simulink model "V2X_Core_SRI_coding_rate_symbol"  (R2023b)
settings: Solver=ode23tb  StartTime=0.0  StopTime=50  MaxStep=1e-2  RelTol=1e-3  AbsTol=1e-3
StopFcn:
  | run('saving.m')
values from neighbouring files (symbols this model uses):
  b = 1.6    [a2024_v2x_matlab_6veh.m]
  m = 2000    [a2024_v2x_matlab_6veh.m]
  mEgo = 1500    [a2024_v2x_matlab_6veh.m]
  Mode = 1    [a2024_v2x_matlab_6veh.m]    (also in v2x_matlab.m; v2x_matlabV2.m; v2x_matlab_6veh.m; v2x_matlab_R.m)
  RefSpeed = 90/3.6    (= 25)    [v2x_matlabV2.m]    (also in v2x_matlab_R.m)
  RelDistThreshold = 300    [v2x_matlabV2.m]    (also in v2x_matlab_R.m)
  s = RandStream("dsfmt19937","Seed",15)    [v2x_matlab.m]
  sampleTime = 0.1    [a2024_v2x_matlab_6veh.m]    (also in v2x_matlab.m; v2x_matlabV2.m; v2x_matlab_6veh.m; v2x_matlab_R.m)
  waypoints = [egoWP(:,2) egoWP(:,1), zeroforwp]    [a2024_v2x_matlab_6veh.m]    (also in misc.m = data.data.ActorSpecifications(1,1).Waypoints(:,[1,2]); v2x_matlab.m = data.data.ActorSpecifications(1,1).Waypoints(:,[1,2]); v2x_matlabV2.m = [5 -1.6 0; v2x_matlab_R.m = [5 -1.6 0)
  ZeroActors = struct(     'ActorID',0,     'Position', [1000 1000 1000],      'Velocity', [0 0 0],      'Roll', 0,      'Pitch', 0,      'Yaw', 0,      'AngularVelocity', [0 0 0])    [v2x_matlabV2.m]    (also in v2x_matlab_R.m)
undefined symbols (not defined in the file or in its folder): Battery, Brakes, Control, DiscIntNeverNeededParam, doppler, Drivetrain, ElectricMotor, Env, FB_flag, Init, SNR_value_list, Vehicle, Wheels
libraries: simulink x45, commofdm x29, commdigbbndam3 x15, commchan3 x14, simulink_extras x13, commcnvcod2 x12, commdigbbndpm3 x11, commblkintrlv2 x10, dspmathops x6, sharedtransform x6, autolibutils x6, autolibsharedcoupling x4
(part 3 of 8)

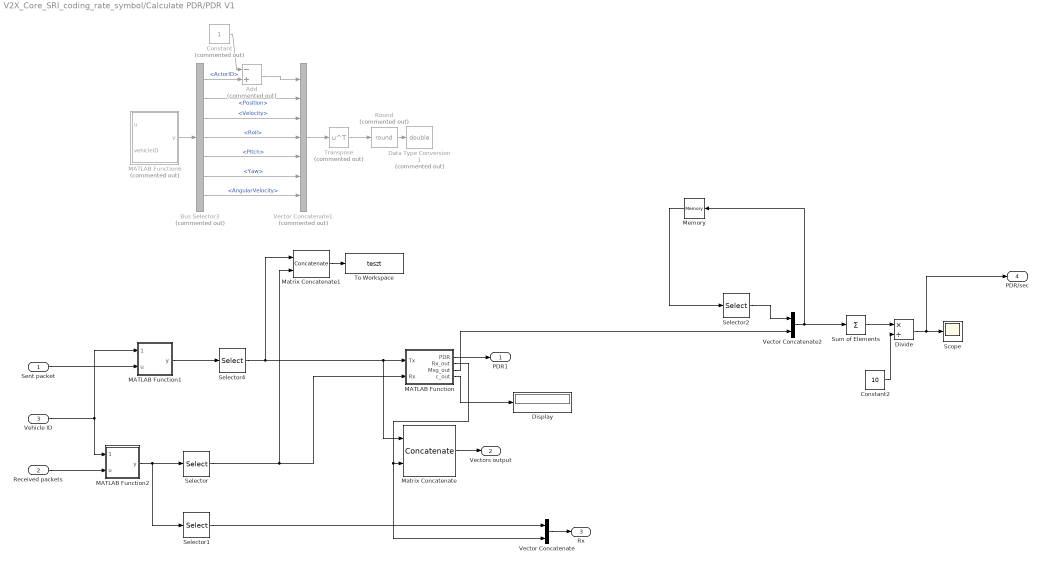
== system V2X_Core_SRI_coding_rate_symbol/Calculate PDR/PDR V1 ==
  Sent packet : Inport
  Received packets : Inport  Port=2
  Vehicle ID : Inport  Port=3
  Add : Sum  Commented=on  Inputs=-+
  Bus Selector3 : BusSelector  Commented=on  OutputSignals=ActorID,Position,Velocity,Roll,Pitch,Yaw,AngularVelocity
  Constant : Constant  Commented=on
  Constant2 : Constant  Value=10
  Data Type Conversion1 : DataTypeConversion  Commented=on  OutDataTypeStr=double  SaturateOnIntegerOverflow=off  RndMeth=Floor
  Display : Display
  Divide : Product  Inputs=*/
  MATLAB Function : MATLAB Function  TreatAsAtomicUnit=on
  MATLAB Function1 : MATLAB Function  TreatAsAtomicUnit=on
  MATLAB Function2 : MATLAB Function  TreatAsAtomicUnit=on
  MATLAB Function6 : MATLAB Function  Commented=on  TreatAsAtomicUnit=on
  Matrix Concatenate : Concatenate  Mode=Multidimensional array  ConcatenateDimension=2
  Matrix Concatenate1 : Concatenate  Mode=Multidimensional array  ConcatenateDimension=2
  Memory : Memory  InitialCondition=zeros(10,1)  InheritSampleTime=on
  Round : Rounding  Commented=on  Operator=round
  Scope : Scope
  Selector : Selector  InputPortWidth=15  IndexOptions=Starting index (dialog)  Indices=3  OutputSizes=13
  Selector1 : Selector  InputPortWidth=15  IndexOptions=Index vector (dialog)  Indices=[1 2]  OutputSizes=13
  Selector2 : Selector  InputPortWidth=10  IndexOptions=Index vector (dialog)  Indices=[2:10]  OutputSizes=1
  Selector4 : Selector  InputPortWidth=15  IndexOptions=Starting index (dialog)  Indices=3  OutputSizes=13
  Sum of Elements : Sum  Inputs=+
  To Workspace : ToWorkspace  VariableName=teszt  SampleTime=-1
  Transpose : Math  Commented=on  Operator=transpose
  Vector Concatenate : Concatenate
  Vector Concatenate1 : Concatenate  Commented=on  NumInputs=7
  Vector Concatenate2 : Concatenate
  PDR1 : Outport
  Vectors output : Outport  Port=2
  Rx : Outport  Port=3
  PDR/sec : Outport  Port=4
  wires:
  MATLAB Function2/1(y) -> Selector1/1, Selector/1
  Received packets/1 -> MATLAB Function2/2(u)
  Selector4/1 -> Matrix Concatenate1/1, Matrix Concatenate/1, MATLAB Function/1(Tx)
  MATLAB Function/1(PDR) -> PDR1/1
  Matrix Concatenate/1 -> Vectors output/1
  Selector/1 -> Matrix Concatenate1/2, MATLAB Function/2(Rx)
  Vehicle ID/1 -> MATLAB Function2/1(Vehicle_ID), MATLAB Function1/1(Vehicle_ID)
  MATLAB Function/2(Rx_out) -> Vector Concatenate/2, Matrix Concatenate/2
  Selector1/1 -> Vector Concatenate/1
  Vector Concatenate/1 -> Rx/1
  MATLAB Function/3(Msg_out) -> Vector Concatenate2/2
  Memory/1 -> Selector2/1
  Selector2/1 -> Vector Concatenate2/1
  Sum of Elements/1 -> Divide/1
  Constant2/1 -> Divide/2
  Divide/1 -> PDR/sec/1, Scope/1
  Vector Concatenate2/1 -> Memory/1, Sum of Elements/1
  Sent packet/1 -> MATLAB Function1/2(u)
  Add/1 -> Vector Concatenate1/1
  Bus Selector3/1 -> Add/2  "<ActorID>"
  Vector Concatenate1/1 -> Transpose/1
  Constant/1 -> Add/1
  Bus Selector3/5 -> Vector Concatenate1/5  "<Pitch>"
  Bus Selector3/2 -> Vector Concatenate1/2  "<Position>"
  Bus Selector3/7 -> Vector Concatenate1/7  "<AngularVelocity>"
  Transpose/1 -> Round/1
  Round/1 -> Data Type Conversion1/1
  Bus Selector3/4 -> Vector Concatenate1/4  "<Roll>"
  Bus Selector3/3 -> Vector Concatenate1/3  "<Velocity>"
  MATLAB Function6/1(y) -> Bus Selector3/1
  Bus Selector3/6 -> Vector Concatenate1/6  "<Yaw>"
  MATLAB Function1/1(y) -> Selector4/1
  MATLAB Function/4(c_out) -> Display/1
  Matrix Concatenate1/1 -> To Workspace/1

== system V2X_Core_SRI_coding_rate_symbol/Calculate PDR/PDR V2 ==
  Sent packet : Inport
  Received packets : Inport  Port=2
  Vehicle ID : Inport  Port=3
  Add : Sum  Commented=on  Inputs=-+
  Bus Selector3 : BusSelector  Commented=on  OutputSignals=ActorID,Position,Velocity,Roll,Pitch,Yaw,AngularVelocity
  Constant : Constant  Commented=on
  Constant2 : Constant  Value=10
  Data Type Conversion1 : DataTypeConversion  Commented=on  OutDataTypeStr=double  SaturateOnIntegerOverflow=off  RndMeth=Floor
  Divide : Product  Inputs=*/
  MATLAB Function : MATLAB Function  TreatAsAtomicUnit=on
  MATLAB Function1 : MATLAB Function  TreatAsAtomicUnit=on
  MATLAB Function2 : MATLAB Function  TreatAsAtomicUnit=on
  MATLAB Function6 : MATLAB Function  Commented=on  TreatAsAtomicUnit=on
  Matrix Concatenate : Concatenate  Mode=Multidimensional array  ConcatenateDimension=2
  Memory : Memory  InitialCondition=zeros(10,1)  InheritSampleTime=on
  Round : Rounding  Commented=on  Operator=round
  Scope : Scope
  Selector : Selector  InputPortWidth=15  IndexOptions=Starting index (dialog)  Indices=3  OutputSizes=13
  Selector1 : Selector  InputPortWidth=15  IndexOptions=Index vector (dialog)  Indices=[1 2]  OutputSizes=13
  Selector2 : Selector  InputPortWidth=10  IndexOptions=Index vector (dialog)  Indices=[2:10]  OutputSizes=1
  Selector4 : Selector  InputPortWidth=15  IndexOptions=Starting index (dialog)  Indices=3  OutputSizes=13
  Sum of Elements : Sum  Inputs=+
  Transpose : Math  Commented=on  Operator=transpose
  Vector Concatenate : Concatenate
  Vector Concatenate1 : Concatenate  Commented=on  NumInputs=7
  Vector Concatenate2 : Concatenate
  PDR2 : Outport
  Vectors output : Outport  Port=2
  Rx : Outport  Port=3
  PDR/sec : Outport  Port=4
  wires:
  MATLAB Function1/1(y) -> Selector4/1
  Bus Selector3/6 -> Vector Concatenate1/6  "<Yaw>"
  MATLAB Function6/1(y) -> Bus Selector3/1
  Bus Selector3/3 -> Vector Concatenate1/3  "<Velocity>"
  Bus Selector3/4 -> Vector Concatenate1/4  "<Roll>"
  Round/1 -> Data Type Conversion1/1
  Transpose/1 -> Round/1
  Bus Selector3/7 -> Vector Concatenate1/7  "<AngularVelocity>"
  Bus Selector3/2 -> Vector Concatenate1/2  "<Position>"
  Bus Selector3/5 -> Vector Concatenate1/5  "<Pitch>"
  Constant/1 -> Add/1
  Vector Concatenate1/1 -> Transpose/1
  Bus Selector3/1 -> Add/2  "<ActorID>"
  Add/1 -> Vector Concatenate1/1
  Sent packet/1 -> MATLAB Function1/2(u)
  Vector Concatenate2/1 -> Sum of Elements/1, Memory/1
  Divide/1 -> Scope/1, PDR/sec/1
  Constant2/1 -> Divide/2
  Sum of Elements/1 -> Divide/1
  Selector2/1 -> Vector Concatenate2/1
  Memory/1 -> Selector2/1
  MATLAB Function/3(Msg_out) -> Vector Concatenate2/2
  Vector Concatenate/1 -> Rx/1
  Selector1/1 -> Vector Concatenate/1
  MATLAB Function/2(Rx_out) -> Matrix Concatenate/2, Vector Concatenate/2
  Vehicle ID/1 -> MATLAB Function2/1(Vehicle_ID), MATLAB Function1/1(Vehicle_ID)
  Selector/1 -> MATLAB Function/2(Rx)
  Matrix Concatenate/1 -> Vectors output/1
  MATLAB Function/1(PDR) -> PDR2/1
  Selector4/1 -> MATLAB Function/1(Tx), Matrix Concatenate/1
  Received packets/1 -> MATLAB Function2/2(u)
  MATLAB Function2/1(y) -> Selector/1, Selector1/1

== system V2X_Core_SRI_coding_rate_symbol/Calculate PDR/PDR V3 ==
  Sent packet : Inport
  Received packets : Inport  Port=2
  Vehicle ID : Inport  Port=3
  Add : Sum  Commented=on  Inputs=-+
  Bus Selector3 : BusSelector  Commented=on  OutputSignals=ActorID,Position,Velocity,Roll,Pitch,Yaw,AngularVelocity
  Constant : Constant  Commented=on
  Constant2 : Constant  Value=10
  Data Type Conversion1 : DataTypeConversion  Commented=on  OutDataTypeStr=double  SaturateOnIntegerOverflow=off  RndMeth=Floor
  Divide : Product  Inputs=*/
  MATLAB Function : MATLAB Function  TreatAsAtomicUnit=on
  MATLAB Function1 : MATLAB Function  TreatAsAtomicUnit=on
  MATLAB Function2 : MATLAB Function  TreatAsAtomicUnit=on
  MATLAB Function6 : MATLAB Function  Commented=on  TreatAsAtomicUnit=on
  Matrix Concatenate : Concatenate  Mode=Multidimensional array  ConcatenateDimension=2
  Memory : Memory  InitialCondition=zeros(10,1)  InheritSampleTime=on
  Round : Rounding  Commented=on  Operator=round
  Scope : Scope
  Selector : Selector  InputPortWidth=15  IndexOptions=Starting index (dialog)  Indices=3  OutputSizes=13
  Selector1 : Selector  InputPortWidth=15  IndexOptions=Index vector (dialog)  Indices=[1 2]  OutputSizes=13
  Selector2 : Selector  InputPortWidth=10  IndexOptions=Index vector (dialog)  Indices=[2:10]  OutputSizes=1
  Selector4 : Selector  InputPortWidth=15  IndexOptions=Starting index (dialog)  Indices=3  OutputSizes=13
  Sum of Elements : Sum  Inputs=+
  Transpose : Math  Commented=on  Operator=transpose
  Vector Concatenate : Concatenate
  Vector Concatenate1 : Concatenate  Commented=on  NumInputs=7
  Vector Concatenate2 : Concatenate
  PDR3 : Outport
  Vectors output : Outport  Port=2
  Rx : Outport  Port=3
  PDR/sec : Outport  Port=4
  wires:
  MATLAB Function2/1(y) -> Selector1/1, Selector/1
  Received packets/1 -> MATLAB Function2/2(u)
  Selector4/1 -> Matrix Concatenate/1, MATLAB Function/1(Tx)
  MATLAB Function/1(PDR) -> PDR3/1
  Matrix Concatenate/1 -> Vectors output/1
  Selector/1 -> MATLAB Function/2(Rx)
  Vehicle ID/1 -> MATLAB Function1/1(Vehicle_ID), MATLAB Function2/1(Vehicle_ID)
  MATLAB Function/2(Rx_out) -> Vector Concatenate/2, Matrix Concatenate/2
  Selector1/1 -> Vector Concatenate/1
  Vector Concatenate/1 -> Rx/1
  MATLAB Function/3(Msg_out) -> Vector Concatenate2/2
  Memory/1 -> Selector2/1
  Selector2/1 -> Vector Concatenate2/1
  Sum of Elements/1 -> Divide/1
  Constant2/1 -> Divide/2
  Divide/1 -> PDR/sec/1, Scope/1
  Vector Concatenate2/1 -> Memory/1, Sum of Elements/1
  Sent packet/1 -> MATLAB Function1/2(u)
  Add/1 -> Vector Concatenate1/1
  Bus Selector3/1 -> Add/2  "<ActorID>"
  Vector Concatenate1/1 -> Transpose/1
  Constant/1 -> Add/1
  Bus Selector3/5 -> Vector Concatenate1/5  "<Pitch>"
  Bus Selector3/2 -> Vector Concatenate1/2  "<Position>"
  Bus Selector3/7 -> Vector Concatenate1/7  "<AngularVelocity>"
  Transpose/1 -> Round/1
  Round/1 -> Data Type Conversion1/1
  Bus Selector3/4 -> Vector Concatenate1/4  "<Roll>"
  Bus Selector3/3 -> Vector Concatenate1/3  "<Velocity>"
  MATLAB Function6/1(y) -> Bus Selector3/1
  Bus Selector3/6 -> Vector Concatenate1/6  "<Yaw>"
  MATLAB Function1/1(y) -> Selector4/1

== system V2X_Core_SRI_coding_rate_symbol/Calculate PDR/PDR V4 ==
  Sent packet : Inport
  Received packets : Inport  Port=2
  Vehicle ID : Inport  Port=3
  Add : Sum  Commented=on  Inputs=-+
  Bus Selector3 : BusSelector  Commented=on  OutputSignals=ActorID,Position,Velocity,Roll,Pitch,Yaw,AngularVelocity
  Constant : Constant  Commented=on
  Constant2 : Constant  Value=10
  Data Type Conversion1 : DataTypeConversion  Commented=on  OutDataTypeStr=double  SaturateOnIntegerOverflow=off  RndMeth=Floor
  Divide : Product  Inputs=*/
  MATLAB Function : MATLAB Function  TreatAsAtomicUnit=on
  MATLAB Function1 : MATLAB Function  TreatAsAtomicUnit=on
  MATLAB Function2 : MATLAB Function  TreatAsAtomicUnit=on
  MATLAB Function6 : MATLAB Function  Commented=on  TreatAsAtomicUnit=on
  Matrix Concatenate : Concatenate  Mode=Multidimensional array  ConcatenateDimension=2
  Memory : Memory  InitialCondition=zeros(10,1)  InheritSampleTime=on
  Round : Rounding  Commented=on  Operator=round
  Scope : Scope
  Selector : Selector  InputPortWidth=15  IndexOptions=Starting index (dialog)  Indices=3  OutputSizes=13
  Selector1 : Selector  InputPortWidth=15  IndexOptions=Index vector (dialog)  Indices=[1 2]  OutputSizes=13
  Selector2 : Selector  InputPortWidth=10  IndexOptions=Index vector (dialog)  Indices=[2:10]  OutputSizes=1
  Selector4 : Selector  InputPortWidth=15  IndexOptions=Starting index (dialog)  Indices=3  OutputSizes=13
  Sum of Elements : Sum  Inputs=+
  Transpose : Math  Commented=on  Operator=transpose
  Vector Concatenate : Concatenate
  Vector Concatenate1 : Concatenate  Commented=on  NumInputs=7
  Vector Concatenate2 : Concatenate
  PDR1 : Outport
  Vectors output : Outport  Port=2
  Rx : Outport  Port=3
  PDR/sec : Outport  Port=4
  wires:
  MATLAB Function1/1(y) -> Selector4/1
  Bus Selector3/6 -> Vector Concatenate1/6  "<Yaw>"
  MATLAB Function6/1(y) -> Bus Selector3/1
  Bus Selector3/3 -> Vector Concatenate1/3  "<Velocity>"
  Bus Selector3/4 -> Vector Concatenate1/4  "<Roll>"
  Round/1 -> Data Type Conversion1/1
  Transpose/1 -> Round/1
  Bus Selector3/7 -> Vector Concatenate1/7  "<AngularVelocity>"
  Bus Selector3/2 -> Vector Concatenate1/2  "<Position>"
  Bus Selector3/5 -> Vector Concatenate1/5  "<Pitch>"
  Constant/1 -> Add/1
  Vector Concatenate1/1 -> Transpose/1
  Bus Selector3/1 -> Add/2  "<ActorID>"
  Add/1 -> Vector Concatenate1/1
  Sent packet/1 -> MATLAB Function1/2(u)
  Vector Concatenate2/1 -> Sum of Elements/1, Memory/1
  Divide/1 -> Scope/1, PDR/sec/1
  Constant2/1 -> Divide/2
  Sum of Elements/1 -> Divide/1
  Selector2/1 -> Vector Concatenate2/1
  Memory/1 -> Selector2/1
  MATLAB Function/3(Msg_out) -> Vector Concatenate2/2
  Vector Concatenate/1 -> Rx/1
  Selector1/1 -> Vector Concatenate/1
  MATLAB Function/2(Rx_out) -> Matrix Concatenate/2, Vector Concatenate/2
  Vehicle ID/1 -> MATLAB Function2/1(Vehicle_ID), MATLAB Function1/1(Vehicle_ID)
  Selector/1 -> MATLAB Function/2(Rx)
  Matrix Concatenate/1 -> Vectors output/1
  MATLAB Function/1(PDR) -> PDR1/1
  Selector4/1 -> MATLAB Function/1(Tx), Matrix Concatenate/1
  Received packets/1 -> MATLAB Function2/2(u)
  MATLAB Function2/1(y) -> Selector/1, Selector1/1

== system V2X_Core_SRI_coding_rate_symbol/Calculate PDR/PDR V5 ==
  Sent packet : Inport
  Received packets : Inport  Port=2
  Vehicle ID : Inport  Port=3
  Add : Sum  Commented=on  Inputs=-+
  Bus Selector3 : BusSelector  Commented=on  OutputSignals=ActorID,Position,Velocity,Roll,Pitch,Yaw,AngularVelocity
  Constant : Constant  Commented=on
  Constant2 : Constant  Value=10
  Data Type Conversion1 : DataTypeConversion  Commented=on  OutDataTypeStr=double  SaturateOnIntegerOverflow=off  RndMeth=Floor
  Divide : Product  Inputs=*/
  MATLAB Function : MATLAB Function  TreatAsAtomicUnit=on
  MATLAB Function1 : MATLAB Function  TreatAsAtomicUnit=on
  MATLAB Function2 : MATLAB Function  TreatAsAtomicUnit=on
  MATLAB Function6 : MATLAB Function  Commented=on  TreatAsAtomicUnit=on
  Matrix Concatenate : Concatenate  Mode=Multidimensional array  ConcatenateDimension=2
  Memory : Memory  InitialCondition=zeros(10,1)  InheritSampleTime=on
  Round : Rounding  Commented=on  Operator=round
  Scope : Scope
  Selector : Selector  InputPortWidth=15  IndexOptions=Starting index (dialog)  Indices=3  OutputSizes=13
  Selector1 : Selector  InputPortWidth=15  IndexOptions=Index vector (dialog)  Indices=[1 2]  OutputSizes=13
  Selector2 : Selector  InputPortWidth=10  IndexOptions=Index vector (dialog)  Indices=[2:10]  OutputSizes=1
  Selector4 : Selector  InputPortWidth=15  IndexOptions=Starting index (dialog)  Indices=3  OutputSizes=13
  Sum of Elements : Sum  Inputs=+
  Transpose : Math  Commented=on  Operator=transpose
  Vector Concatenate : Concatenate
  Vector Concatenate1 : Concatenate  Commented=on  NumInputs=7
  Vector Concatenate2 : Concatenate
  PDR1 : Outport
  Vectors output : Outport  Port=2
  Rx : Outport  Port=3
  PDR/sec : Outport  Port=4
  wires:
  MATLAB Function2/1(y) -> Selector1/1, Selector/1
  Received packets/1 -> MATLAB Function2/2(u)
  Selector4/1 -> Matrix Concatenate/1, MATLAB Function/1(Tx)
  MATLAB Function/1(PDR) -> PDR1/1
  Matrix Concatenate/1 -> Vectors output/1
  Selector/1 -> MATLAB Function/2(Rx)
  Vehicle ID/1 -> MATLAB Function1/1(Vehicle_ID), MATLAB Function2/1(Vehicle_ID)
  MATLAB Function/2(Rx_out) -> Vector Concatenate/2, Matrix Concatenate/2
  Selector1/1 -> Vector Concatenate/1
  Vector Concatenate/1 -> Rx/1
  MATLAB Function/3(Msg_out) -> Vector Concatenate2/2
  Memory/1 -> Selector2/1
  Selector2/1 -> Vector Concatenate2/1
  Sum of Elements/1 -> Divide/1
  Constant2/1 -> Divide/2
  Divide/1 -> PDR/sec/1, Scope/1
  Vector Concatenate2/1 -> Memory/1, Sum of Elements/1
  Sent packet/1 -> MATLAB Function1/2(u)
  Add/1 -> Vector Concatenate1/1
  Bus Selector3/1 -> Add/2  "<ActorID>"
  Vector Concatenate1/1 -> Transpose/1
  Constant/1 -> Add/1
  Bus Selector3/5 -> Vector Concatenate1/5  "<Pitch>"
  Bus Selector3/2 -> Vector Concatenate1/2  "<Position>"
  Bus Selector3/7 -> Vector Concatenate1/7  "<AngularVelocity>"
  Transpose/1 -> Round/1
  Round/1 -> Data Type Conversion1/1
  Bus Selector3/4 -> Vector Concatenate1/4  "<Roll>"
  Bus Selector3/3 -> Vector Concatenate1/3  "<Velocity>"
  MATLAB Function6/1(y) -> Bus Selector3/1
  Bus Selector3/6 -> Vector Concatenate1/6  "<Yaw>"
  MATLAB Function1/1(y) -> Selector4/1

== system V2X_Core_SRI_coding_rate_symbol/Calculate PDR/PDR V6 ==
  Sent packet : Inport
  Received packets : Inport  Port=2
  Vehicle ID : Inport  Port=3
  Add : Sum  Commented=on  Inputs=-+
  Bus Selector3 : BusSelector  Commented=on  OutputSignals=ActorID,Position,Velocity,Roll,Pitch,Yaw,AngularVelocity
  Constant : Constant  Commented=on
  Constant2 : Constant  Value=10
  Data Type Conversion1 : DataTypeConversion  Commented=on  OutDataTypeStr=double  SaturateOnIntegerOverflow=off  RndMeth=Floor
  Divide : Product  Inputs=*/
  MATLAB Function : MATLAB Function  TreatAsAtomicUnit=on
  MATLAB Function1 : MATLAB Function  TreatAsAtomicUnit=on
  MATLAB Function2 : MATLAB Function  TreatAsAtomicUnit=on
  MATLAB Function6 : MATLAB Function  Commented=on  TreatAsAtomicUnit=on
  Matrix Concatenate : Concatenate  Mode=Multidimensional array  ConcatenateDimension=2
  Memory : Memory  InitialCondition=zeros(10,1)  InheritSampleTime=on
  Round : Rounding  Commented=on  Operator=round
  Scope : Scope
  Selector : Selector  InputPortWidth=15  IndexOptions=Starting index (dialog)  Indices=3  OutputSizes=13
  Selector1 : Selector  InputPortWidth=15  IndexOptions=Index vector (dialog)  Indices=[1 2]  OutputSizes=13
  Selector2 : Selector  InputPortWidth=10  IndexOptions=Index vector (dialog)  Indices=[2:10]  OutputSizes=1
  Selector4 : Selector  InputPortWidth=15  IndexOptions=Starting index (dialog)  Indices=3  OutputSizes=13
  Sum of Elements : Sum  Inputs=+
  Transpose : Math  Commented=on  Operator=transpose
  Vector Concatenate : Concatenate
  Vector Concatenate1 : Concatenate  Commented=on  NumInputs=7
  Vector Concatenate2 : Concatenate
  PDR1 : Outport
  Vectors output : Outport  Port=2
  Rx : Outport  Port=3
  PDR/sec : Outport  Port=4
  wires:
  MATLAB Function1/1(y) -> Selector4/1
  Bus Selector3/6 -> Vector Concatenate1/6  "<Yaw>"
  MATLAB Function6/1(y) -> Bus Selector3/1
  Bus Selector3/3 -> Vector Concatenate1/3  "<Velocity>"
  Bus Selector3/4 -> Vector Concatenate1/4  "<Roll>"
  Round/1 -> Data Type Conversion1/1
  Transpose/1 -> Round/1
  Bus Selector3/7 -> Vector Concatenate1/7  "<AngularVelocity>"
  Bus Selector3/2 -> Vector Concatenate1/2  "<Position>"
  Bus Selector3/5 -> Vector Concatenate1/5  "<Pitch>"
  Constant/1 -> Add/1
  Vector Concatenate1/1 -> Transpose/1
  Bus Selector3/1 -> Add/2  "<ActorID>"
  Add/1 -> Vector Concatenate1/1
  Sent packet/1 -> MATLAB Function1/2(u)
  Vector Concatenate2/1 -> Sum of Elements/1, Memory/1
  Divide/1 -> Scope/1, PDR/sec/1
  Constant2/1 -> Divide/2
  Sum of Elements/1 -> Divide/1
  Selector2/1 -> Vector Concatenate2/1
  Memory/1 -> Selector2/1
  MATLAB Function/3(Msg_out) -> Vector Concatenate2/2
  Vector Concatenate/1 -> Rx/1
  Selector1/1 -> Vector Concatenate/1
  MATLAB Function/2(Rx_out) -> Matrix Concatenate/2, Vector Concatenate/2
  Vehicle ID/1 -> MATLAB Function2/1(Vehicle_ID), MATLAB Function1/1(Vehicle_ID)
  Selector/1 -> MATLAB Function/2(Rx)
  Matrix Concatenate/1 -> Vectors output/1
  MATLAB Function/1(PDR) -> PDR1/1
  Selector4/1 -> MATLAB Function/1(Tx), Matrix Concatenate/1
  Received packets/1 -> MATLAB Function2/2(u)
  MATLAB Function2/1(y) -> Selector/1, Selector1/1

== system V2X_Core_SRI_coding_rate_symbol/DSRC/Queue ==
  Actors : Inport
  Bus Selector : BusSelector  OutputSignals=Actor1,Actor2,Actor3,Actor4,Actor5,Actor6
  Counter Limited : simulink/Sources/Counter Limited  uplimit=4  tsamp=0.01
  Merge : Merge  Inputs=6
  Scope1 : Scope
  Switch Case : SwitchCase  CaseConditions={0,1,2,3,4,5}  ShowDefaultCase=off
  Switch Case Action Subsystem : Subsystem  TreatAsAtomicUnit=on
  Switch Case Action Subsystem1 : Subsystem  TreatAsAtomicUnit=on
  Switch Case Action Subsystem2 : Subsystem  TreatAsAtomicUnit=on
  Switch Case Action Subsystem3 : Subsystem  TreatAsAtomicUnit=on
  Switch Case Action Subsystem4 : Subsystem  TreatAsAtomicUnit=on
  Switch Case Action Subsystem5 : Subsystem  TreatAsAtomicUnit=on
  Actor : Outport
  wires:
  Switch Case/4 -> Switch Case Action Subsystem3/Action
  Switch Case Action Subsystem5/1(Out1) -> Merge/6
  Counter Limited/1 -> Switch Case/1, Scope1/1  "Control"
  Switch Case/2 -> Switch Case Action Subsystem1/Action
  Switch Case Action Subsystem3/1(Out1) -> Merge/4
  Switch Case Action Subsystem4/1(Out1) -> Merge/5
  Switch Case/1 -> Switch Case Action Subsystem/Action
  Switch Case/6 -> Switch Case Action Subsystem5/Action
  Switch Case Action Subsystem2/1(Out1) -> Merge/3
  Switch Case/3 -> Switch Case Action Subsystem2/Action
  Switch Case/5 -> Switch Case Action Subsystem4/Action
  Switch Case Action Subsystem1/1(Out1) -> Merge/2
  Bus Selector/2 -> Switch Case Action Subsystem1/1(Actor1)  "<Actor2>"
  Bus Selector/3 -> Switch Case Action Subsystem2/1(In1)  "<Actor3>"
  Bus Selector/4 -> Switch Case Action Subsystem3/1(In1)  "<Actor4>"
  Bus Selector/5 -> Switch Case Action Subsystem4/1(In1)  "<Actor5>"
  Bus Selector/6 -> Switch Case Action Subsystem5/1(In1)  "<Actor6>"
  Actors/1 -> Bus Selector/1
  Bus Selector/1 -> Switch Case Action Subsystem/1(Actor1)  "<Actor1>"
  Merge/1 -> Actor/1
  Switch Case Action Subsystem/1(Actor) -> Merge/1

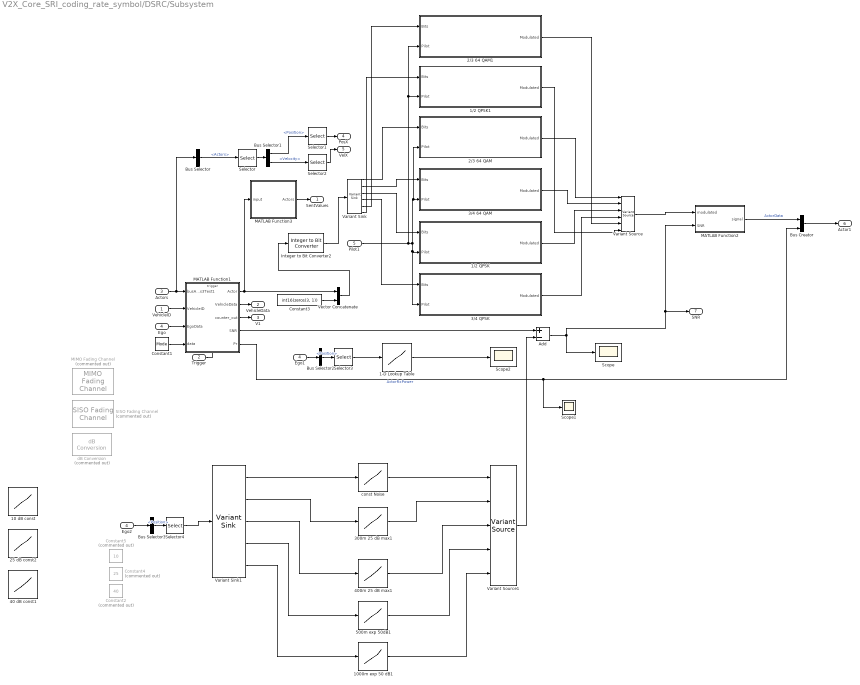
== system V2X_Core_SRI_coding_rate_symbol/DSRC/Subsystem ==
  VehicleID : Inport
  Trigger : Inport  Port=2
  Actors : Inport  Port=3
  Ego : Inport  Port=4
  Pilot1 : Inport  Port=5
  " 10 dB const" : Lookup_n-D  NumberOfTableDimensions=1  BreakpointsForDimension1=[0 100 200 300 400 500 600 700 800 900 1000]  Table=[10 10 10 10 10 10 10 10 10 10 10]  InternalRulePriority=Speed  RndMeth=Simplest
  " 25 dB const2" : Lookup_n-D  NumberOfTableDimensions=1  BreakpointsForDimension1=[0 100 200 300 400 500 600 700 800 900 1000]  Table=[25 25 25 25 25 25 25 25 25 25 25]  InternalRulePriority=Speed  RndMeth=Simplest
  " 40 dB const1" : Lookup_n-D  NumberOfTableDimensions=1  BreakpointsForDimension1=[0 100 200 300 400 500 600 700 800 900 1000]  Table=[40 40 40 40 40 40 40 40 40 40 40]  InternalRulePriority=Speed  RndMeth=Simplest
  1-D Lookup Table : Lookup_n-D  NumberOfTableDimensions=1  BreakpointsForDimension1=[0 100 200 300 400 500 600 700 800 900 1000]  Table=[5 10 15 20 15 10 5 0 0 0 0]  InternalRulePriority=Speed  RndMeth=Simplest
  1/2 QPSK : Subsystem  TreatAsAtomicUnit=on
  1/2 QPSK1 : Subsystem  TreatAsAtomicUnit=on
  1000m exp 50 dB1 : Lookup_n-D  NumberOfTableDimensions=1  BreakpointsForDimension1=[0;100;200;300;400;500;600;700;800;900;1000;2000]  Table=[1;1;1.58;2.51;3.98;6.31;10;15.85;25.12;39.81;50;50]  InternalRulePriority=Speed  RndMeth=Simplest
  2/3 64 QAM : Subsystem  TreatAsAtomicUnit=on
  2/3 64 QAM1 : Subsystem  TreatAsAtomicUnit=on
  3/4 64 QAM : Subsystem  TreatAsAtomicUnit=on
  3/4 QPSK : Subsystem  TreatAsAtomicUnit=on
  300m 25 dB max1 : Lookup_n-D  NumberOfTableDimensions=1  BreakpointsForDimension1=[0 100 200 300 400 500 600 700 800 900 1000]  Table=[10 15 20 25 20 15 10 5 0 0 0]  InternalRulePriority=Speed  RndMeth=Simplest
  400m 25 dB max1 : Lookup_n-D  NumberOfTableDimensions=1  BreakpointsForDimension1=[0 100 200 300 400 500 600 700 800 900 1000]  Table=[5 10 15 20 25 20 15 10 5 0 0]  InternalRulePriority=Speed  RndMeth=Simplest
  500m exp 50dB1 : Lookup_n-D  NumberOfTableDimensions=1  BreakpointsForDimension1=[0;100;200;300;400;500;600;700;800;900;1000;2000]  Table=[1;1;1.58;2.51;3.98;6.31;10;15.85;25.12;39.81;50;50]  InternalRulePriority=Speed  RndMeth=Simplest
  Add : Sum  Inputs=+-
  Bus Creator : BusCreator  Inputs=2
  Bus Selector : BusSelector  OutputSignals=Actors
  Bus Selector1 : BusSelector  OutputSignals=Position,Velocity
  Bus Selector2 : BusSelector  OutputSignals=Position
  Bus Selector3 : BusSelector  OutputSignals=Position
  Constant1 : Constant  Value=Mode
  Constant2 : Constant  Commented=on  Value=40
  Constant3 : Constant  Value=int16(zeros(3, 1))
  Constant4 : Constant  Commented=on  Value=25
  Constant5 : Constant  Commented=on  Value=10
  Ego1 : InportShadow  Port=4
  Ego2 : InportShadow  Port=4
  Integer to Bit Converter2 : simulink/Logic and Bit Operations/Integer to Bit Converter  nbits=16  signedInputValues=Signed  bitOrder=MSB first  outDtype=int16
  MATLAB Function1 : MATLAB Function  TreatAsAtomicUnit=on
  MATLAB Function2 : MATLAB Function  TreatAsAtomicUnit=on
  MATLAB Function3 : MATLAB Function  TreatAsAtomicUnit=on  SystemSampleTime=0.01
  MIMO Fading Channel : commchan3/MIMO Fading Channel  Commented=on  InheritSampleRate=on  SampleRate=1  PathDelays=0  AveragePathGains=0  NormalizePathGains=on  FadingDistribution=Rayleigh  KFactor=3  DirectPathDopplerShift=0  DirectPathInitialPhase=0  MaximumDopplerShift=0.001  DopplerSpectrum=doppler('Jakes')  SpatialCorrelationSpecification=None  SpatialCorrelationMatrix=[1 0 0 0; 0 1 0 0; 0 0 1 0; 0 0 0 1]  NumTransmitAntennas=1  NumReceiveAntennas=1  TransmitCorrelationMatrix=[1 0; 0 1]  ReceiveCorrelationMatrix=[1 0; 0 1]  AntennaSelection=Off  NormalizeChannelOutputs=on  PathGainsOutputPort=off  SimulateUsing=Interpreted execution  FadingTechnique=Filtered Gaussian noise  NumSinusoids=48  InitialTimeSource=Property  InitialTime=0  RandomStream=mt19937ar with seed  Seed=73  Visualization=Off  AntennaPairsToDisplay=[ 1, 1 ]  PathsForDopplerDisplay=1  SamplesToDisplay=25%
  SISO Fading Channel : commchan3/SISO Fading Channel  Commented=on  InheritSampleRate=off  SampleRate=5.9e9  PathDelays=0  AveragePathGains=0  NormalizePathGains=on  FadingDistribution=Rayleigh  KFactor=3  DirectPathDopplerShift=0  DirectPathInitialPhase=0  MaximumDopplerShift=0.001  DopplerSpectrum=doppler('Jakes')  RandomStream=mt19937ar with seed  Seed=73  PathGainsOutputPort=off  ChannelFilterDelayOutputPort=off  SimulateUsing=Interpreted execution  Visualization=Off  PathsForDopplerDisplay=1  SamplesToDisplay=25%
  Scope : Scope
  Scope1 : Scope
  Scope2 : Scope
  Selector : Selector  InputPortWidth=1  IndexOptions=Index vector (dialog)  Indices=1  OutputSizes=1
  Selector1 : Selector  InputPortWidth=3  IndexOptions=Index vector (dialog)  Indices=1  OutputSizes=1
  Selector2 : Selector  InputPortWidth=3  IndexOptions=Index vector (dialog)  Indices=1  OutputSizes=1
  Selector3 : Selector  InputPortWidth=3  IndexOptions=Index vector (dialog)  Indices=[1]  OutputSizes=1
  Selector4 : Selector  InputPortWidth=3  IndexOptions=Index vector (dialog)  Indices=[1]  OutputSizes=1
  Variant Sink : VariantSink
  Variant Sink1 : VariantSink
  Variant Source : VariantSource
  Variant Source1 : VariantSource
  Vector Concatenate : Concatenate
  const Noise : Lookup_n-D  NumberOfTableDimensions=1  BreakpointsForDimension1=[0 100 200 300 400 500 600 700 800 900 1000]  Table=SNR_value_list  InternalRulePriority=Speed  RndMeth=Simplest
  dB Conversion : dspmathops/dB Conversion  Commented=on  dBtype=dB  intype=Amplitude  R=1  fuzz=off
      settings: LibrarySourceBlock=commutil2/dB Conversion
  SentValues : Outport
  VehicleData : Outport  Port=2
  V1 : Outport  Port=3
  PosX : Outport  Port=4
  VelX : Outport  Port=5
  Actor1 : Outport  Port=6
  SNR : Outport  Port=7
  wires:
  MATLAB Function1/1(Actor) -> MATLAB Function3/1(input), Vector Concatenate/1
  Ego/1 -> MATLAB Function1/3(EgoData)
  Actors/1 -> Bus Selector/1, MATLAB Function1/1(busActors3Test1)
  VehicleID/1 -> MATLAB Function1/2(VehicleID)
  MATLAB Function1/2(VehicleData) -> VehicleData/1
  MATLAB Function1/3(counter_out) -> V1/1
  Trigger/1 -> MATLAB Function1/Trigger
  MATLAB Function1/5(Pr) -> Scope1/1, Bus Creator/2  "ActorRxPower"
  MATLAB Function1/4(SNR) -> Add/1
  Add/1 -> SNR/1, MATLAB Function2/2(SNR), Scope/1
  Selector1/1 -> PosX/1
  Bus Selector/1 -> Selector/1  "<Actors>"
  Selector/1 -> Bus Selector1/1
  Bus Selector1/1 -> Selector1/1  "<Position>"
  Bus Selector1/2 -> Selector2/1  "<Velocity>"
  Selector2/1 -> VelX/1
  Variant Sink/4 -> 3/4 QPSK/1(Bits)
  Pilot1/1 -> 1/2 QPSK1/2(Pilot), 2/3 64 QAM1/2(Pilot), 3/4 QPSK/2(Pilot), 1/2 QPSK/2(Pilot), 2/3 64 QAM/2(Pilot), 3/4 64 QAM/2(Pilot)
  Integer to Bit Converter2/1 -> Variant Sink/1
  3/4 QPSK/1(Modulated) -> Variant Source/4
  3/4 64 QAM/1(Modulated) -> Variant Source/2
  Variant Sink/2 -> 3/4 64 QAM/1(Bits)
  Bus Creator/1 -> Actor1/1
  MATLAB Function3/1(Actors) -> SentValues/1
  Constant1/1 -> MATLAB Function1/4(data)
  1-D Lookup Table/1 -> Scope2/1
  Constant3/1 -> Vector Concatenate/2
  Vector Concatenate/1 -> Integer to Bit Converter2/1
  Variant Source/1 -> MATLAB Function2/1(modulated)
  MATLAB Function2/1(signal) -> Bus Creator/1  "ActorData"
  Variant Sink/3 -> 1/2 QPSK/1(Bits)
  Variant Sink/1 -> 2/3 64 QAM/1(Bits)
  1/2 QPSK/1(Modulated) -> Variant Source/3
  2/3 64 QAM/1(Modulated) -> Variant Source/1
  Ego1/1 -> Bus Selector2/1
  Bus Selector2/1 -> Selector3/1  "<Position>"
  Selector3/1 -> 1-D Lookup Table/1
  Bus Selector3/1 -> Selector4/1  "<Position>"
  Ego2/1 -> Bus Selector3/1
  const Noise/1 -> Variant Source1/1
  300m 25 dB max1/1 -> Variant Source1/2
  400m 25 dB max1/1 -> Variant Source1/3
  500m exp 50dB1/1 -> Variant Source1/4
  1000m exp 50 dB1/1 -> Variant Source1/5
  Selector4/1 -> Variant Sink1/1
  Variant Source1/1 -> Add/2
  Variant Sink/5 -> 2/3 64 QAM1/1(Bits)
  2/3 64 QAM1/1(Modulated) -> Variant Source/5
  Variant Sink/6 -> 1/2 QPSK1/1(Bits)
  1/2 QPSK1/1(Modulated) -> Variant Source/6
  Variant Sink1/1 -> const Noise/1
  Variant Sink1/2 -> 300m 25 dB max1/1
  Variant Sink1/3 -> 400m 25 dB max1/1
  Variant Sink1/4 -> 500m exp 50dB1/1
  Variant Sink1/5 -> 1000m exp 50 dB1/1

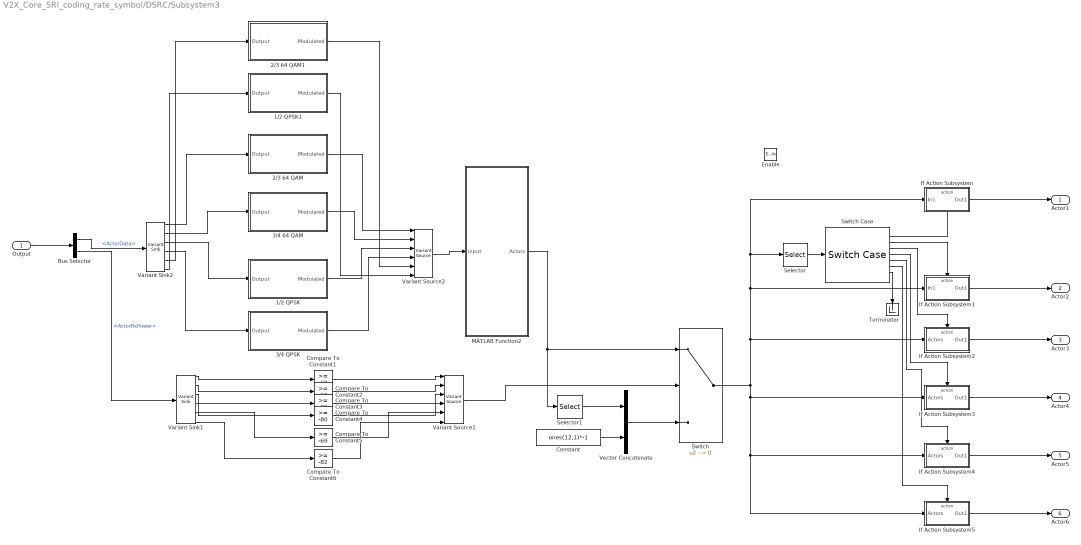
== system V2X_Core_SRI_coding_rate_symbol/DSRC/Subsystem3 ==
  Output : Inport
  Enable : EnablePort
  1/2 QPSK : Subsystem  TreatAsAtomicUnit=on
  1/2 QPSK1 : Subsystem  TreatAsAtomicUnit=on
  2/3 64 QAM : Subsystem  TreatAsAtomicUnit=on
  2/3 64 QAM1 : Subsystem  TreatAsAtomicUnit=on
  3/4 64 QAM : Subsystem  TreatAsAtomicUnit=on
  3/4 QPSK : Subsystem  TreatAsAtomicUnit=on
  Bus Selector : BusSelector  OutputSignals=ActorData,ActorRxPower
  Compare To Constant1 : simulink/Logic and Bit Operations/Compare To Constant  relop=>=  const=-69  OutDataTypeStr=boolean
  Compare To Constant2 : simulink/Logic and Bit Operations/Compare To Constant  relop=>=  const=-68  OutDataTypeStr=boolean
  Compare To Constant3 : simulink/Logic and Bit Operations/Compare To Constant  relop=>=  const=-82  OutDataTypeStr=boolean
  Compare To Constant4 : simulink/Logic and Bit Operations/Compare To Constant  relop=>=  const=-80  OutDataTypeStr=boolean
  Compare To Constant5 : simulink/Logic and Bit Operations/Compare To Constant  relop=>=  const=-69  OutDataTypeStr=boolean
  Compare To Constant6 : simulink/Logic and Bit Operations/Compare To Constant  relop=>=  const=-82  OutDataTypeStr=boolean
  Constant : Constant  Value=ones(12,1)*-1
  If Action Subsystem : Subsystem  TreatAsAtomicUnit=on
  If Action Subsystem1 : Subsystem  TreatAsAtomicUnit=on
  If Action Subsystem2 : Subsystem  TreatAsAtomicUnit=on
  If Action Subsystem3 : Subsystem  TreatAsAtomicUnit=on
  If Action Subsystem4 : Subsystem  TreatAsAtomicUnit=on
  If Action Subsystem5 : Subsystem  TreatAsAtomicUnit=on
  MATLAB Function2 : MATLAB Function  TreatAsAtomicUnit=on  SystemSampleTime=0.01
  Selector : Selector  InputPortWidth=15  IndexOptions=Index vector (dialog)  Indices=[3]  OutputSizes=1
  Selector1 : Selector  InputPortWidth=15  IndexOptions=Index vector (dialog)  Indices=[1:3]  OutputSizes=1
  Switch : Switch  Criteria=u2 ~= 0  SaturateOnIntegerOverflow=off  InputSameDT=off
  Switch Case : SwitchCase  CaseConditions={1,2,3,4,5,6}
  Terminator : Terminator
  Variant Sink1 : VariantSink
      settings: AllowZeroVariantControls=on
  Variant Sink2 : VariantSink
  Variant Source1 : VariantSource
  Variant Source2 : VariantSource
  Vector Concatenate : Concatenate
  Actor1 : Outport
  Actor2 : Outport  Port=2
  Actor3 : Outport  Port=3
  Actor4 : Outport  Port=4
  Actor5 : Outport  Port=5
  Actor6 : Outport  Port=6
  wires:
  Selector/1 -> Switch Case/1
  Switch Case/1 -> If Action Subsystem/Action
  If Action Subsystem/1(Out1) -> Actor1/1
  If Action Subsystem1/1(Out1) -> Actor2/1
  Switch Case/2 -> If Action Subsystem1/Action
  Variant Source2/1 -> MATLAB Function2/1(input)
  If Action Subsystem2/1(Out1) -> Actor3/1
  Switch Case/3 -> If Action Subsystem2/Action
  If Action Subsystem3/1(Out1) -> Actor4/1
  Switch/1 -> If Action Subsystem/1(In1), Selector/1, If Action Subsystem1/1(In1), If Action Subsystem2/1(Actors), If Action Subsystem5/1(Actors), If Action Subsystem4/1(Actors), If Action Subsystem3/1(Actors)
  Switch Case/4 -> If Action Subsystem3/Action
  Switch Case/7 -> Terminator/1
  If Action Subsystem4/1(Out1) -> Actor5/1
  Switch Case/5 -> If Action Subsystem4/Action
  If Action Subsystem5/1(Out1) -> Actor6/1
  Switch Case/6 -> If Action Subsystem5/Action
  Variant Sink2/2 -> 3/4 64 QAM/1(Output)
  Variant Sink2/4 -> 3/4 QPSK/1(Output)
  3/4 64 QAM/1(Modulated) -> Variant Source2/2
  3/4 QPSK/1(Modulated) -> Variant Source2/4
  MATLAB Function2/1(Actors) -> Selector1/1, Switch/1
  Output/1 -> Bus Selector/1
  Selector1/1 -> Vector Concatenate/1
  Constant/1 -> Vector Concatenate/2
  Vector Concatenate/1 -> Switch/3
  Bus Selector/1 -> Variant Sink2/1  "<ActorData>"
  Bus Selector/2 -> Variant Sink1/1  "<ActorRxPower>"
  Variant Source1/1 -> Switch/2
  Variant Sink2/1 -> 2/3 64 QAM/1(Output)
  Variant Sink2/3 -> 1/2 QPSK/1(Output)
  2/3 64 QAM/1(Modulated) -> Variant Source2/1
  1/2 QPSK/1(Modulated) -> Variant Source2/3
  Compare To Constant4/1 -> Variant Source1/4
  Compare To Constant3/1 -> Variant Source1/3
  Compare To Constant2/1 -> Variant Source1/2
  Compare To Constant1/1 -> Variant Source1/1
  Variant Sink1/1 -> Compare To Constant1/1
  Variant Sink1/2 -> Compare To Constant2/1
  Variant Sink1/3 -> Compare To Constant3/1
  Variant Sink1/4 -> Compare To Constant4/1
  Variant Sink1/5 -> Compare To Constant5/1
  Compare To Constant5/1 -> Variant Source1/5
  Variant Sink2/5 -> 2/3 64 QAM1/1(Output)
  2/3 64 QAM1/1(Modulated) -> Variant Source2/5
  Variant Sink2/6 -> 1/2 QPSK1/1(Output)
  1/2 QPSK1/1(Modulated) -> Variant Source2/6
  Variant Sink1/6 -> Compare To Constant6/1
  Compare To Constant6/1 -> Variant Source1/6

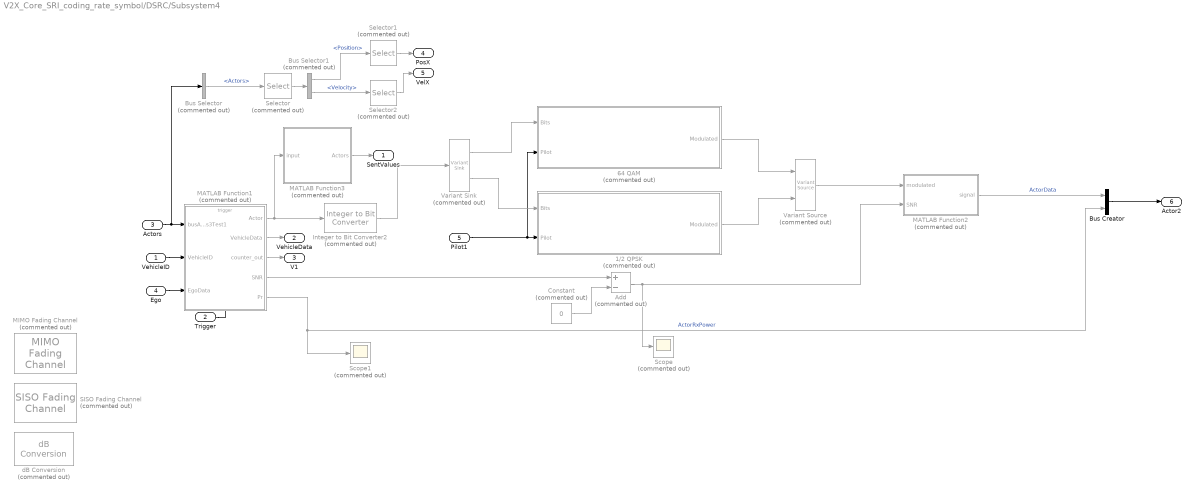
== system V2X_Core_SRI_coding_rate_symbol/DSRC/Subsystem4 ==
  VehicleID : Inport
  Trigger : Inport  Port=2
  Actors : Inport  Port=3
  Ego : Inport  Port=4
  Pilot1 : Inport  Port=5
  1/2 QPSK : Subsystem  Commented=on  TreatAsAtomicUnit=on
  64 QAM : Subsystem  Commented=on  TreatAsAtomicUnit=on
  Add : Sum  Commented=on  Inputs=+-
  Bus Creator : BusCreator  Inputs=2
  Bus Selector : BusSelector  Commented=on  OutputSignals=Actors
  Bus Selector1 : BusSelector  Commented=on  OutputSignals=Position,Velocity
  Constant : Constant  Commented=on  Value=0
  Integer to Bit Converter2 : simulink/Logic and Bit Operations/Integer to Bit Converter  Commented=on  nbits=16  signedInputValues=Signed  bitOrder=MSB first  outDtype=boolean
  MATLAB Function1 : MATLAB Function  Commented=on  TreatAsAtomicUnit=on
  MATLAB Function2 : MATLAB Function  Commented=on  TreatAsAtomicUnit=on
  MATLAB Function3 : MATLAB Function  Commented=on  TreatAsAtomicUnit=on  SystemSampleTime=0.01
  MIMO Fading Channel : commchan3/MIMO Fading Channel  Commented=on  InheritSampleRate=on  SampleRate=1  PathDelays=0  AveragePathGains=0  NormalizePathGains=on  FadingDistribution=Rayleigh  KFactor=3  DirectPathDopplerShift=0  DirectPathInitialPhase=0  MaximumDopplerShift=0.001  DopplerSpectrum=doppler('Jakes')  SpatialCorrelationSpecification=None  SpatialCorrelationMatrix=[1 0 0 0; 0 1 0 0; 0 0 1 0; 0 0 0 1]  NumTransmitAntennas=1  NumReceiveAntennas=1  TransmitCorrelationMatrix=[1 0; 0 1]  ReceiveCorrelationMatrix=[1 0; 0 1]  AntennaSelection=Off  NormalizeChannelOutputs=on  PathGainsOutputPort=off  SimulateUsing=Interpreted execution  FadingTechnique=Filtered Gaussian noise  NumSinusoids=48  InitialTimeSource=Property  InitialTime=0  RandomStream=mt19937ar with seed  Seed=73  Visualization=Off  AntennaPairsToDisplay=[ 1, 1 ]  PathsForDopplerDisplay=1  SamplesToDisplay=25%
  SISO Fading Channel : commchan3/SISO Fading Channel  Commented=on  InheritSampleRate=off  SampleRate=5.9e9  PathDelays=0  AveragePathGains=0  NormalizePathGains=on  FadingDistribution=Rayleigh  KFactor=3  DirectPathDopplerShift=0  DirectPathInitialPhase=0  MaximumDopplerShift=0.001  DopplerSpectrum=doppler('Jakes')  RandomStream=mt19937ar with seed  Seed=73  PathGainsOutputPort=off  ChannelFilterDelayOutputPort=off  SimulateUsing=Interpreted execution  Visualization=Off  PathsForDopplerDisplay=1  SamplesToDisplay=25%
  Scope : Scope  Commented=on
  Scope1 : Scope  Commented=on
  Selector : Selector  Commented=on  InputPortWidth=1  IndexOptions=Index vector (dialog)  Indices=1  OutputSizes=1
  Selector1 : Selector  Commented=on  InputPortWidth=3  IndexOptions=Index vector (dialog)  Indices=1  OutputSizes=1
  Selector2 : Selector  Commented=on  InputPortWidth=3  IndexOptions=Index vector (dialog)  Indices=1  OutputSizes=1
  Variant Sink : VariantSink  Commented=on
  Variant Source : VariantSource  Commented=on
  dB Conversion : dspmathops/dB Conversion  Commented=on  dBtype=dB  intype=Amplitude  R=1  fuzz=off
      settings: LibrarySourceBlock=commutil2/dB Conversion
  SentValues : Outport
  VehicleData : Outport  Port=2
  V1 : Outport  Port=3
  PosX : Outport  Port=4
  VelX : Outport  Port=5
  Actor2 : Outport  Port=6
  wires:
  MATLAB Function3/1(Actors) -> SentValues/1
  Bus Creator/1 -> Actor2/1
  MATLAB Function2/1(signal) -> Bus Creator/1  "ActorData"
  Constant/1 -> Add/2
  Variant Sink/1 -> 64 QAM/1(Bits)
  64 QAM/1(Modulated) -> Variant Source/1
  1/2 QPSK/1(Modulated) -> Variant Source/2
  Variant Source/1 -> MATLAB Function2/1(modulated)
  Integer to Bit Converter2/1 -> Variant Sink/1
  Pilot1/1 -> 1/2 QPSK/2(Pilot), 64 QAM/2(Pilot)
  Variant Sink/2 -> 1/2 QPSK/1(Bits)
  Selector2/1 -> VelX/1
  Bus Selector1/2 -> Selector2/1  "<Velocity>"
  Bus Selector1/1 -> Selector1/1  "<Position>"
  Selector/1 -> Bus Selector1/1
  Bus Selector/1 -> Selector/1  "<Actors>"
  Selector1/1 -> PosX/1
  Add/1 -> Scope/1, MATLAB Function2/2(SNR)
  MATLAB Function1/4(SNR) -> Add/1
  MATLAB Function1/5(Pr) -> Scope1/1, Bus Creator/2  "ActorRxPower"
  Trigger/1 -> MATLAB Function1/Trigger
  MATLAB Function1/3(counter_out) -> V1/1
  MATLAB Function1/2(VehicleData) -> VehicleData/1
  VehicleID/1 -> MATLAB Function1/2(VehicleID)
  Actors/1 -> MATLAB Function1/1(busActors3Test1), Bus Selector/1
  Ego/1 -> MATLAB Function1/3(EgoData)
  MATLAB Function1/1(Actor) -> Integer to Bit Converter2/1, MATLAB Function3/1(input)

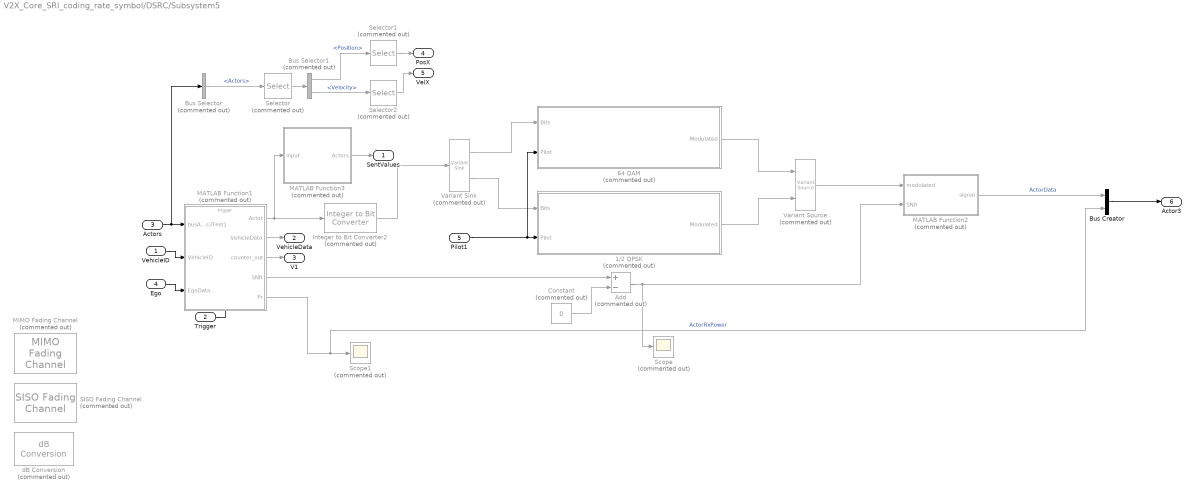
== system V2X_Core_SRI_coding_rate_symbol/DSRC/Subsystem5 ==
  VehicleID : Inport
  Trigger : Inport  Port=2
  Actors : Inport  Port=3
  Ego : Inport  Port=4
  Pilot1 : Inport  Port=5
  1/2 QPSK : Subsystem  Commented=on  TreatAsAtomicUnit=on
  64 QAM : Subsystem  Commented=on  TreatAsAtomicUnit=on
  Add : Sum  Commented=on  Inputs=+-
  Bus Creator : BusCreator  Inputs=2
  Bus Selector : BusSelector  Commented=on  OutputSignals=Actors
  Bus Selector1 : BusSelector  Commented=on  OutputSignals=Position,Velocity
  Constant : Constant  Commented=on  Value=0
  Integer to Bit Converter2 : simulink/Logic and Bit Operations/Integer to Bit Converter  Commented=on  nbits=16  signedInputValues=Signed  bitOrder=MSB first  outDtype=boolean
  MATLAB Function1 : MATLAB Function  Commented=on  TreatAsAtomicUnit=on
  MATLAB Function2 : MATLAB Function  Commented=on  TreatAsAtomicUnit=on
  MATLAB Function3 : MATLAB Function  Commented=on  TreatAsAtomicUnit=on  SystemSampleTime=0.01
  MIMO Fading Channel : commchan3/MIMO Fading Channel  Commented=on  InheritSampleRate=on  SampleRate=1  PathDelays=0  AveragePathGains=0  NormalizePathGains=on  FadingDistribution=Rayleigh  KFactor=3  DirectPathDopplerShift=0  DirectPathInitialPhase=0  MaximumDopplerShift=0.001  DopplerSpectrum=doppler('Jakes')  SpatialCorrelationSpecification=None  SpatialCorrelationMatrix=[1 0 0 0; 0 1 0 0; 0 0 1 0; 0 0 0 1]  NumTransmitAntennas=1  NumReceiveAntennas=1  TransmitCorrelationMatrix=[1 0; 0 1]  ReceiveCorrelationMatrix=[1 0; 0 1]  AntennaSelection=Off  NormalizeChannelOutputs=on  PathGainsOutputPort=off  SimulateUsing=Interpreted execution  FadingTechnique=Filtered Gaussian noise  NumSinusoids=48  InitialTimeSource=Property  InitialTime=0  RandomStream=mt19937ar with seed  Seed=73  Visualization=Off  AntennaPairsToDisplay=[ 1, 1 ]  PathsForDopplerDisplay=1  SamplesToDisplay=25%
  SISO Fading Channel : commchan3/SISO Fading Channel  Commented=on  InheritSampleRate=off  SampleRate=5.9e9  PathDelays=0  AveragePathGains=0  NormalizePathGains=on  FadingDistribution=Rayleigh  KFactor=3  DirectPathDopplerShift=0  DirectPathInitialPhase=0  MaximumDopplerShift=0.001  DopplerSpectrum=doppler('Jakes')  RandomStream=mt19937ar with seed  Seed=73  PathGainsOutputPort=off  ChannelFilterDelayOutputPort=off  SimulateUsing=Interpreted execution  Visualization=Off  PathsForDopplerDisplay=1  SamplesToDisplay=25%
  Scope : Scope  Commented=on
  Scope1 : Scope  Commented=on
  Selector : Selector  Commented=on  InputPortWidth=1  IndexOptions=Index vector (dialog)  Indices=1  OutputSizes=1
  Selector1 : Selector  Commented=on  InputPortWidth=3  IndexOptions=Index vector (dialog)  Indices=1  OutputSizes=1
  Selector2 : Selector  Commented=on  InputPortWidth=3  IndexOptions=Index vector (dialog)  Indices=1  OutputSizes=1
  Variant Sink : VariantSink  Commented=on
  Variant Source : VariantSource  Commented=on
  dB Conversion : dspmathops/dB Conversion  Commented=on  dBtype=dB  intype=Amplitude  R=1  fuzz=off
      settings: LibrarySourceBlock=commutil2/dB Conversion
  SentValues : Outport
  VehicleData : Outport  Port=2
  V1 : Outport  Port=3
  PosX : Outport  Port=4
  VelX : Outport  Port=5
  Actor3 : Outport  Port=6
  wires:
  MATLAB Function1/1(Actor) -> MATLAB Function3/1(input), Integer to Bit Converter2/1
  Ego/1 -> MATLAB Function1/3(EgoData)
  Actors/1 -> Bus Selector/1, MATLAB Function1/1(busActors3Test1)
  VehicleID/1 -> MATLAB Function1/2(VehicleID)
  MATLAB Function1/2(VehicleData) -> VehicleData/1
  MATLAB Function1/3(counter_out) -> V1/1
  Trigger/1 -> MATLAB Function1/Trigger
  MATLAB Function1/5(Pr) -> Bus Creator/2, Scope1/1  "ActorRxPower"
  MATLAB Function1/4(SNR) -> Add/1
  Add/1 -> MATLAB Function2/2(SNR), Scope/1
  Selector1/1 -> PosX/1
  Bus Selector/1 -> Selector/1  "<Actors>"
  Selector/1 -> Bus Selector1/1
  Bus Selector1/1 -> Selector1/1  "<Position>"
  Bus Selector1/2 -> Selector2/1  "<Velocity>"
  Selector2/1 -> VelX/1
  Variant Sink/2 -> 1/2 QPSK/1(Bits)
  Pilot1/1 -> 64 QAM/2(Pilot), 1/2 QPSK/2(Pilot)
  Integer to Bit Converter2/1 -> Variant Sink/1
  Variant Source/1 -> MATLAB Function2/1(modulated)
  1/2 QPSK/1(Modulated) -> Variant Source/2
  64 QAM/1(Modulated) -> Variant Source/1
  Variant Sink/1 -> 64 QAM/1(Bits)
  Constant/1 -> Add/2
  MATLAB Function2/1(signal) -> Bus Creator/1  "ActorData"
  Bus Creator/1 -> Actor3/1
  MATLAB Function3/1(Actors) -> SentValues/1

== system V2X_Core_SRI_coding_rate_symbol/DSRC/Subsystem6 ==
  VehicleID : Inport
  Trigger : Inport  Port=2
  Actors : Inport  Port=3
  Ego : Inport  Port=4
  Pilot1 : Inport  Port=5
  1/2 QPSK : Subsystem  Commented=on  TreatAsAtomicUnit=on
  64 QAM : Subsystem  Commented=on  TreatAsAtomicUnit=on
  Add : Sum  Commented=on  Inputs=+-
  Bus Creator : BusCreator  Inputs=2
  Bus Selector : BusSelector  Commented=on  OutputSignals=Actors
  Bus Selector1 : BusSelector  Commented=on  OutputSignals=Position,Velocity
  Constant : Constant  Commented=on  Value=0
  Integer to Bit Converter2 : simulink/Logic and Bit Operations/Integer to Bit Converter  Commented=on  nbits=16  signedInputValues=Signed  bitOrder=MSB first  outDtype=boolean
  MATLAB Function1 : MATLAB Function  Commented=on  TreatAsAtomicUnit=on
  MATLAB Function2 : MATLAB Function  Commented=on  TreatAsAtomicUnit=on
  MATLAB Function3 : MATLAB Function  Commented=on  TreatAsAtomicUnit=on  SystemSampleTime=0.01
  MIMO Fading Channel : commchan3/MIMO Fading Channel  Commented=on  InheritSampleRate=on  SampleRate=1  PathDelays=0  AveragePathGains=0  NormalizePathGains=on  FadingDistribution=Rayleigh  KFactor=3  DirectPathDopplerShift=0  DirectPathInitialPhase=0  MaximumDopplerShift=0.001  DopplerSpectrum=doppler('Jakes')  SpatialCorrelationSpecification=None  SpatialCorrelationMatrix=[1 0 0 0; 0 1 0 0; 0 0 1 0; 0 0 0 1]  NumTransmitAntennas=1  NumReceiveAntennas=1  TransmitCorrelationMatrix=[1 0; 0 1]  ReceiveCorrelationMatrix=[1 0; 0 1]  AntennaSelection=Off  NormalizeChannelOutputs=on  PathGainsOutputPort=off  SimulateUsing=Interpreted execution  FadingTechnique=Filtered Gaussian noise  NumSinusoids=48  InitialTimeSource=Property  InitialTime=0  RandomStream=mt19937ar with seed  Seed=73  Visualization=Off  AntennaPairsToDisplay=[ 1, 1 ]  PathsForDopplerDisplay=1  SamplesToDisplay=25%
  SISO Fading Channel : commchan3/SISO Fading Channel  Commented=on  InheritSampleRate=off  SampleRate=5.9e9  PathDelays=0  AveragePathGains=0  NormalizePathGains=on  FadingDistribution=Rayleigh  KFactor=3  DirectPathDopplerShift=0  DirectPathInitialPhase=0  MaximumDopplerShift=0.001  DopplerSpectrum=doppler('Jakes')  RandomStream=mt19937ar with seed  Seed=73  PathGainsOutputPort=off  ChannelFilterDelayOutputPort=off  SimulateUsing=Interpreted execution  Visualization=Off  PathsForDopplerDisplay=1  SamplesToDisplay=25%
  Scope : Scope  Commented=on
  Scope1 : Scope  Commented=on
  Selector : Selector  Commented=on  InputPortWidth=1  IndexOptions=Index vector (dialog)  Indices=1  OutputSizes=1
  Selector1 : Selector  Commented=on  InputPortWidth=3  IndexOptions=Index vector (dialog)  Indices=1  OutputSizes=1
  Selector2 : Selector  Commented=on  InputPortWidth=3  IndexOptions=Index vector (dialog)  Indices=1  OutputSizes=1
  Variant Sink : VariantSink  Commented=on
  Variant Source : VariantSource  Commented=on
  dB Conversion : dspmathops/dB Conversion  Commented=on  dBtype=dB  intype=Amplitude  R=1  fuzz=off
      settings: LibrarySourceBlock=commutil2/dB Conversion
  SentValues : Outport
  VehicleData : Outport  Port=2
  V1 : Outport  Port=3
  PosX : Outport  Port=4
  VelX : Outport  Port=5
  Actor4 : Outport  Port=6
  wires:
  MATLAB Function3/1(Actors) -> SentValues/1
  Bus Creator/1 -> Actor4/1
  MATLAB Function2/1(signal) -> Bus Creator/1  "ActorData"
  Constant/1 -> Add/2
  Variant Sink/1 -> 64 QAM/1(Bits)
  64 QAM/1(Modulated) -> Variant Source/1
  1/2 QPSK/1(Modulated) -> Variant Source/2
  Variant Source/1 -> MATLAB Function2/1(modulated)
  Integer to Bit Converter2/1 -> Variant Sink/1
  Pilot1/1 -> 1/2 QPSK/2(Pilot), 64 QAM/2(Pilot)
  Variant Sink/2 -> 1/2 QPSK/1(Bits)
  Selector2/1 -> VelX/1
  Bus Selector1/2 -> Selector2/1  "<Velocity>"
  Bus Selector1/1 -> Selector1/1  "<Position>"
  Selector/1 -> Bus Selector1/1
  Bus Selector/1 -> Selector/1  "<Actors>"
  Selector1/1 -> PosX/1
  Add/1 -> Scope/1, MATLAB Function2/2(SNR)
  MATLAB Function1/4(SNR) -> Add/1
  MATLAB Function1/5(Pr) -> Scope1/1, Bus Creator/2  "ActorRxPower"
  Trigger/1 -> MATLAB Function1/Trigger
  MATLAB Function1/3(counter_out) -> V1/1
  MATLAB Function1/2(VehicleData) -> VehicleData/1
  VehicleID/1 -> MATLAB Function1/2(VehicleID)
  Actors/1 -> MATLAB Function1/1(busActors3Test1), Bus Selector/1
  Ego/1 -> MATLAB Function1/3(EgoData)
  MATLAB Function1/1(Actor) -> Integer to Bit Converter2/1, MATLAB Function3/1(input)
